simulink model "TTR_mdl"  (Simulink 8.1)
settings: Solver=ode3  StartTime=0.0  StopTime=100  FixedStep=Ts  MaxStep=Ts  RelTol=1e-3
InitFcn:
  | TTR_mdl_Initialization;
model workspace: external: MAT-File C:\Users\Kostas\Documents\GitHub\robust_mpc\Verified_Examples\TTR\TTR_mdl_workspace.mat (data not in the file)
values from neighbouring files (symbols this model uses):
  Damping = [damping_phi; damping_theta; damping_psi; damping_x; damping_y; damping_z]    [TTR_Initialization.m]    (also in TTR_mdl_Dynamics.m = block.DialogPrm(3).Data; TTR_mdl_Initialization.m = cell2struct( num2cell(Damping_arr), {'phi','theta','psi','x'; TTR_mdl_workspace.mat = )
  Drag = block.DialogPrm(4).Data    [TTR_mdl_Dynamics.m]    (also in TTR_mdl_Initialization.m = cell2struct( num2cell(Drag_arr), {'a','b'}, 1 ); TTR_mdl_workspace.mat = )
  F_0 = block.DialogPrm(5).Data    [TTR_mdl_Dynamics.m]    (also in TTR_mdl_Initialization.m = solve('d_RL_x*(FL_0+FR_0)=d_T_x*FT_0','FR_0+FL_0+FT_0=m_B*g'; TTR_mdl_workspace.mat = )
  g = 9.81    [TTR_Initialization.m]    (also in TTR_mdl_Dynamics.m = TTR_mdl_Properties.g; TTR_mdl_Initialization.m)
  LQR_phi = [92.7047477254 36.0877897074 4.11128151093 0.0597844255793]    [TTR_mdl_workspace.mat]
  m_B = 2.350    (= 2.35)    [TTR_Initialization.m]    (also in TTR_mdl_Dynamics.m = TTR_mdl_Properties.m_B; TTR_mdl_Initialization.m)
  PolyGT_U2A = [0.002181661564993 0.0]    [TTR_Initialization.m]    (also in TTR_mdl_Initialization.m; TTR_mdl_workspace.mat = [0.00218166156499 0])
  PolyRL_U2R = (PolyR_U2R + PolyL_U2R)/2    [TTR_mdl_Initialization.m]    (also in TTR_mdl_workspace.mat = [7.59051955434 1446.30527598])
  PolyT_U2R = 1.0e+03*[0.007882307894585   1.022799157396815]    [TTR_Initialization.m]    (also in TTR_mdl_Initialization.m; TTR_mdl_workspace.mat = [7.88230789458 1022.7991574])
  Rotor_Properties = cell2struct( num2cell(Rotor_Properties_arr), {'C_T_RL_trim','C_T_RL_prop','C_T_T_trim','C_T_T_prop'}, 1 )    [TTR_mdl_Initialization.m]    (also in TTR_mdl_workspace.mat = )
  tf_RL0_ss = idss(tf_RL0_p,'SSParameterization','Canonical')    [TTR_mdl_Initialization.m]
  tf_RL_ss = idss(tf_RL_p,'SSParameterization','Canonical')    [TTR_mdl_Initialization.m]
  tf_S_den = tf_S.den{1}    [TTR_mdl_Initialization.m]    (also in TTR_mdl_workspace.mat = [1 30])
  tf_S_num = tf_S.num{1}    [TTR_mdl_Initialization.m]    (also in TTR_mdl_workspace.mat = [0 30])
  tf_T0_ss = idss(tf_T0_p,'SSParameterization','Canonical')    [TTR_mdl_Initialization.m]
  tf_T_ss = idss(tf_T_p,'SSParameterization','Canonical')    [TTR_mdl_Initialization.m]
  Ts_slow = 0.250    (= 0.25)    [TTR_Initialization.m]    (also in TTR_mdl_Initialization.m = TTR_RobustMPC.Xdir.Ts; TTR_mdl_workspace.mat = 0.2)
  TTR_mdl_Properties = block.DialogPrm(1).Data    [TTR_mdl_Dynamics.m]    (also in TTR_mdl_Initialization.m = cell2struct( num2cell(TTR_mdl_Properties_arr), {'m_B','g','I; TTR_mdl_workspace.mat = )
  TTR_mdl_Properties_arr = [ m_B; g; Ixx; Iyy; Izz; Ixy; Ixz; Iyz; d_RL_x; d_T_x; d_RL_y; d_T_y; d_RL_z; d_T_z; h_RL; h_T; rho; w_chord; w_span; w_ac_x; w_ac_y ]    [TTR_mdl_Initialization.m]    (also in TTR_mdl_workspace.mat = [2.35 9.81 0.057748141 0.025379458 0.074710979 0 0 0 0.05461)
  TTR_RobustMPC =     [RobustMPC_TTRctrls.mat]    (also in RobustMPC_TTRctrls_INFnorm.mat)
  Wing_Properties = block.DialogPrm(2).Data    [TTR_mdl_Dynamics.m]    (also in TTR_mdl_Initialization.m = struct(                  'a_vect' , a_vect ,                ; TTR_mdl_workspace.mat = )
libraries: simulink_extras x5, Robust_MPC_Library x3
settings Model: Creator=babis  LastModifiedBy=Kostas
settings SolverCC: AutoInsertRateTranBlk=on  InsertRTBMode=Always
settings DataIOCC: SaveOutput=off  SaveState=on
settings OptimizationCC: InlineParams=on  InlineInvariantSignals=on  StateBitsets=on  DataBitsets=on  UseTempVars=on  ZeroExternalMemoryAtStartup=off  ZeroInternalMemoryAtStartup=off  NoFixptDivByZeroProtection=on  OptimizeModelRefInitCode=on  LifeSpan=1
settings DebuggingCC: AlgebraicLoopMsg=none  SolverPrmCheckMsg=none  UnconnectedInputMsg=none  UnconnectedOutputMsg=none  UnconnectedLineMsg=none
settings HardwareCC: ProdIntDivRoundTo=Floor  ProdEndianess=LittleEndian  ProdHWDeviceType=Generic->Custom
settings SFSimCC: SimUserIncludeDirs=/home/atum/workspace/Matlab/src  SimBuildMode=sf_nonincremental_build
settings RTWCC: SystemTargetFile=ert.tlc  TLCOptions=-p0  GenCodeOnly=on  TemplateMakefile=ert_default_tmf  Description=Real-Time Workshop Embedded Coder  GenerateReport=on  RTWVerbose=off  ProcessScript=ert_make_rtw_hook  RTWUseSimCustomCode=on  CustomInclude=/home/atum/workspace/Matlab/src  IncludeHyperlinkInReport=on  LaunchReport=on
settings CodeAppCC: ForceParamTrailComments=on  IgnoreCustomStorageClasses=off  SimulinkDataObjDesc=on  CustomSymbolStrGlobalVar=rt$N$M  CustomSymbolStrType=$N$M  CustomSymbolStrFcn=$N$M$F  CustomSymbolStrMacro=$N$M  InsertBlockDesc=on  InternalIdentifier=Classic
settings ERTTargetCC: CodeReplacementLibrary=ISO_C  MultiwordLength=2048  GenerateSampleERTMain=on  IncludeMdlTerminateFcn=off  SuppressErrorStatus=on  SupportAbsoluteTime=off  SupportNonFinite=off  SupportComplex=off  InlinedParameterPlacement=NonHierarchical  RootIOFormat=Structure reference  ERTCustomFileTemplate=example_file_process.tlc  ConvertIfToSwitch=off  SuppressUnreachableDefaultCases=off

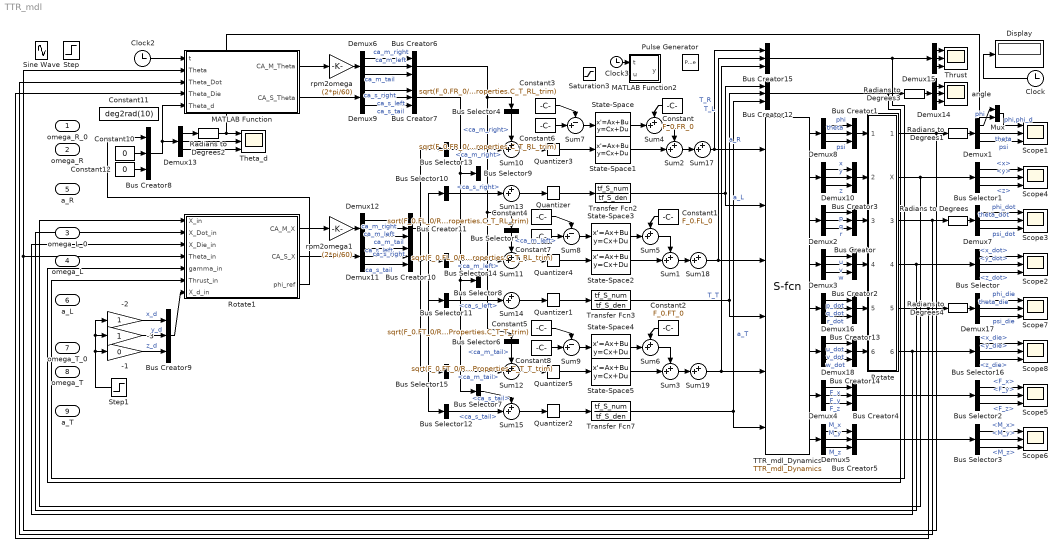
== system TTR_mdl ==
  omega_R_0 : Inport
  omega_R : Inport  Port=2
  omega_L_0 : Inport  Port=3
  omega_L : Inport  Port=4
  a_R : Inport  Port=5
  a_L : Inport  Port=6
  omega_T_0 : Inport  Port=7
  omega_T : Inport  Port=8
  a_T : Inport  Port=9
  -1 : Gain  Gain=0
  -2 : Gain
  -3 : Gain
  Bus Creator{,1..15} (16 alike) : BusCreator  Inputs=3
  Bus Selector : BusSelector  OutputSignals=x_dot,y_dot,z_dot
  Bus Selector1 : BusSelector  OutputSignals=x,y,z
  Bus Selector10 : BusSelector  OutputSignals=ca_s_right
  Bus Selector11 : BusSelector  OutputSignals=ca_s_left
  Bus Selector12 : BusSelector  OutputSignals=ca_s_tail
  Bus Selector13 : BusSelector  OutputSignals=ca_m_right
  Bus Selector14 : BusSelector  OutputSignals=ca_m_left
  Bus Selector15 : BusSelector  OutputSignals=ca_m_tail
  Bus Selector16 : BusSelector  OutputSignals=x_die,y_die,z_die
  Bus Selector2 : BusSelector  OutputSignals=F_x,F_y,F_z
  Bus Selector3 : BusSelector  OutputSignals=M_x,M_y,M_z
  Bus Selector4 : BusSelector  OutputSignals=ca_m_right
  Bus Selector5 : BusSelector  OutputSignals=ca_m_left
  Bus Selector6 : BusSelector  OutputSignals=ca_m_tail
  Bus Selector7 : BusSelector  OutputSignals=ca_s_tail
  Bus Selector8 : BusSelector  OutputSignals=ca_s_left
  Bus Selector9 : BusSelector  OutputSignals=ca_s_right
  Clock : Clock
  Clock2 : Clock
  Clock3 : Clock
  Constant : Constant  Value=F_0.FR_0
  Constant1 : Constant  Value=F_0.FL_0
  Constant10 : Constant  Value=0
  Constant11 : Constant  Value=deg2rad(10)
  Constant12 : Constant  Value=0
  Constant2 : Constant  Value=F_0.FT_0
  Constant3 : Constant  Value=sqrt(F_0.FR_0/Rotor_Properties.C_T_RL_trim)
  Constant4 : Constant  Value=sqrt(F_0.FL_0/Rotor_Properties.C_T_RL_trim)
  Constant5 : Constant  Value=sqrt(F_0.FT_0/Rotor_Properties.C_T_T_trim)
  Constant6 : Constant  Value=sqrt(F_0.FR_0/Rotor_Properties.C_T_RL_trim)
  Constant7 : Constant  Value=sqrt(F_0.FL_0/Rotor_Properties.C_T_RL_trim)
  Constant8 : Constant  Value=sqrt(F_0.FT_0/Rotor_Properties.C_T_T_trim)
  Demux{1..18} (18 alike) : Demux  Outputs=3
  Display : Display
  MATLAB Function : MATLAB Function  TreatAsAtomicUnit=on
  MATLAB Function2 : MATLAB Function  TreatAsAtomicUnit=on
  Mux : Mux  Inputs=2
  Pulse Generator : DiscretePulseGenerator  PulseType=Time based  Amplitude=0.1  Period=10  PulseWidth=50
  Quantizer : Quantizer  QuantizationInterval=deg2rad(0.5)
  Quantizer1 : Quantizer  QuantizationInterval=deg2rad(0.5)
  Quantizer2 : Quantizer  QuantizationInterval=deg2rad(0.5)
  Quantizer3 : Quantizer  QuantizationInterval=(1/(2*pi/60))*(1/PolyRL_U2R(1))
  Quantizer4 : Quantizer  QuantizationInterval=(1/(2*pi/60))*(1/PolyRL_U2R(1))
  Quantizer5 : Quantizer  QuantizationInterval=(1/(2*pi/60))*(1/PolyT_U2R(1))
  Radians to Degrees{,1..4} (5 alike) : simulink_extras/Transformations/Radians to Degrees
  Rotate : Subsystem
  Rotate1 : Subsystem
  Saturation3 : Saturate  UpperLimit=deg2rad(15)  LowerLimit=-deg2rad(15)
  Scope{1..8} (8 alike) : Scope  NumInputPorts=3
      Scope1 settings: TimeRange=100  YMin=-3.5~-0.225~-0.05  YMax=3.5~0.35~0.225  SaveName=Theta
      Scope2 settings: TimeRange=100  YMin=-0.004~0.005~0.0255  YMax=0.003~0.025~0.0285  SaveName=X_Dot
      Scope3 settings: TimeRange=100  YMin=-45~-0.25~-0.06  YMax=-30~0.25~0.02  SaveName=Theta_Dot
      Scope4 settings: TimeRange=100  YMin=5.55112e-17~0.1~-0.0225  YMax=1.5~2~0.015  SaveName=X
      Scope5 settings: TimeRange=100  YMin=-1~-2~-0.8  YMax=2.5~3~0.6000000000000001  SaveName=F
      Scope6 settings: TimeRange=100  YMin=-0.1~-0.01~-0.015  YMax=0.1~0.015~0.01  SaveName=M
      Scope7 settings: TimeRange=100  YMin=-100~-30~-10  YMax=100~30~10  SaveName=Theta_Die
      Scope8 settings: TimeRange=100  YMin=0~0~-5  YMax=100~800~5  SaveName=X_Die
  Sine Wave : Sin  Amplitude=deg2rad(10)  Frequency=0.1*(60/(2*pi))  SampleTime=0
  State-Space : StateSpace  A=tf_RL0_ss.A  B=tf_RL0_ss.B  C=tf_RL0_ss.C  D=tf_RL0_ss.D  X0=[0;0]
  State-Space1 : StateSpace  A=tf_RL_ss.A  B=tf_RL_ss.B  C=tf_RL_ss.C  D=tf_RL_ss.D  X0=[0;0]
  State-Space2 : StateSpace  A=tf_RL_ss.A  B=tf_RL_ss.B  C=tf_RL_ss.C  D=tf_RL_ss.D  X0=[0;0]
  State-Space3 : StateSpace  A=tf_RL0_ss.A  B=tf_RL0_ss.B  C=tf_RL0_ss.C  D=tf_RL0_ss.D  X0=[0;0]
  State-Space4 : StateSpace  A=tf_T0_ss.A  B=tf_T0_ss.B  C=tf_T0_ss.C  D=tf_T0_ss.D  X0=[0;0]
  State-Space5 : StateSpace  A=tf_T_ss.A  B=tf_T_ss.B  C=tf_T_ss.C  D=tf_T_ss.D  X0=[0;0]
  Step : Step  Time=50  After=[-1;-1;1]  SampleTime=0
  Step1 : Step  SampleTime=0
  Sum{1..6,10..15,17..19} (15 alike) : Sum  Inputs=++|
  Sum7 : Sum  Inputs=-+|
  Sum8 : Sum  Inputs=-+|
  Sum9 : Sum  Inputs=-+|
  TTR_mdl_Dynamics : M-S-Function  FunctionName=TTR_mdl_Dynamics  Parameters=TTR_mdl_Properties,Wing_Properties,Damping,Drag,F_0  mask{TTR_mdl_Properties=TTR_mdl_Properties, Wing_Properties=Wing_Properties, Damping=Damping, Drag=Drag, F_0=F_0}
      mask Display:
      | port_label('input',1,'T_R')
      | port_label('input',2,'a_R')
      | port_label('input',3,'T_L')
      | port_label('input',4,'a_L')
      | port_label('input',5,'T_T')
      | port_label('input',6,'a_T')
      | 
      | port_label('output',1,'Theta')
      | port_label('output',2,'X')
      | port_label('output',3,'Omega')
      | port_label('output',4,'U')
      | 
      | port_label('output',5,'Omega_Dot')
      | port_label('output',6,'U_Dot')
      | 
      | port_label('output',7,'F_tot')
      | port_label('output',8,'M_tot')
  Theta_d : Scope  NumInputPorts=3
      settings: TimeRange=100  YMin=0.248709~-9525~-5  YMax=0.274889~-9300~5  SaveName=Theta_d
  Thrust : Scope  NumInputPorts=3
      settings: TimeRange=16  YMin=10.2759~10.2759~1.516  YMax=11.3575~11.3575~1.529  SaveName=F_A
  Transfer Fcn2 : TransferFcn  Numerator=tf_S_num  Denominator=tf_S_den
  Transfer Fcn3 : TransferFcn  Numerator=tf_S_num  Denominator=tf_S_den
  Transfer Fcn7 : TransferFcn  Numerator=tf_S_num  Denominator=tf_S_den
  angle : Scope  NumInputPorts=3
      settings: TimeRange=100  YMin=14.25~14.25~-1  YMax=15.75~15.75~1  SaveName=Gamma
  rpm2omega : Gain  Gain=(2*pi/60)
  rpm2omega1 : Gain  Gain=(2*pi/60)
  wires:
  Transfer Fcn2/1 -> TTR_mdl_Dynamics/2, Bus Creator12/1  "a_R"
  Transfer Fcn3/1 -> TTR_mdl_Dynamics/4, Bus Creator12/2  "a_L"
  Radians to Degrees/1 -> Demux7/1
  Clock/1 -> Display/1
  Demux7/1 -> Scope3/1  "phi_dot"
  Demux7/2 -> Scope3/2  "theta_dot"
  Demux7/3 -> Scope3/3  "psi_dot"
  Radians to Degrees1/1 -> Demux1/1
  Demux1/2 -> Scope1/2  "theta"
  Demux1/3 -> Scope1/3  "psi"
  Bus Selector1/1 -> Scope4/1  "<x>"
  Bus Selector1/2 -> Scope4/2  "<y>"
  Bus Selector1/3 -> Scope4/3  "<z>"
  Bus Selector3/1 -> Scope6/1  "<M_x>"
  Bus Selector3/2 -> Scope6/2  "<M_y>"
  Bus Selector3/3 -> Scope6/3  "<M_z>"
  Transfer Fcn7/1 -> TTR_mdl_Dynamics/6, Bus Creator12/3  "a_T"
  State-Space1/1 -> Sum2/2
  State-Space2/1 -> Sum1/2
  State-Space5/1 -> Sum3/2
  State-Space/1 -> Sum4/2
  Sum4/1 -> Sum2/1
  Constant/1 -> Sum4/1
  Constant1/1 -> Sum5/1
  State-Space3/1 -> Sum5/2
  Sum5/1 -> Sum1/1
  Constant2/1 -> Sum6/1
  State-Space4/1 -> Sum6/2
  Sum6/1 -> Sum3/1
  Sum7/1 -> State-Space/1
  Constant3/1 -> Sum7/1
  Constant4/1 -> Sum8/1
  Sum8/1 -> State-Space3/1
  Constant5/1 -> Sum9/1
  Sum9/1 -> State-Space4/1
  Constant6/1 -> Sum7/2
  Constant7/1 -> Sum8/2
  Constant8/1 -> Sum9/2
  Demux2/1 -> Bus Creator/1  "p"
  Demux2/2 -> Bus Creator/2  "q"
  Demux2/3 -> Bus Creator/3  "r"
  Demux8/1 -> Bus Creator1/1  "phi"
  Demux8/2 -> Bus Creator1/2  "theta"
  Demux8/3 -> Bus Creator1/3  "psi"
  Demux3/1 -> Bus Creator2/1  "u"
  Demux3/2 -> Bus Creator2/2  "v"
  Demux3/3 -> Bus Creator2/3  "w"
  Demux10/1 -> Bus Creator3/1  "x"
  Demux10/2 -> Bus Creator3/2  "y"
  Bus Selector/1 -> Scope2/1  "<x_dot>"
  Bus Selector/2 -> Scope2/2  "<y_dot>"
  Bus Selector/3 -> Scope2/3  "<z_dot>"
  Demux4/1 -> Bus Creator4/1  "F_x"
  Demux4/2 -> Bus Creator4/2  "F_y"
  Demux4/3 -> Bus Creator4/3  "F_z"
  Bus Creator4/1 -> Bus Selector2/1
  Bus Selector2/1 -> Scope5/1  "<F_x>"
  Bus Selector2/2 -> Scope5/2  "<F_y>"
  Bus Selector2/3 -> Scope5/3  "<F_z>"
  Demux5/1 -> Bus Creator5/1  "M_x"
  Demux5/2 -> Bus Creator5/2  "M_y"
  Demux5/3 -> Bus Creator5/3  "M_z"
  Bus Creator5/1 -> Bus Selector3/1
  Demux6/1 -> Bus Creator6/1  "ca_m_right"
  Demux6/2 -> Bus Creator6/2  "ca_m_left"
  Demux6/3 -> Bus Creator6/3  "ca_m_tail"
  Sum10/1 -> Quantizer3/1
  Sum11/1 -> Quantizer4/1
  Sum12/1 -> Quantizer5/1
  MATLAB Function/1(CA_M_Theta) -> rpm2omega/1
  rpm2omega/1 -> Demux6/1
  Demux9/1 -> Bus Creator7/1  "ca_s_right"
  Demux9/2 -> Bus Creator7/2  "ca_s_left"
  Demux9/3 -> Bus Creator7/3  "ca_s_tail"
  MATLAB Function/2(CA_S_Theta) -> Demux9/1
  Bus Creator6/1 -> Bus Selector5/1, Bus Selector6/1, Bus Selector4/1
  Bus Selector4/1 -> Sum10/1  "<ca_m_right>"
  Bus Selector5/1 -> Sum11/1  "<ca_m_left>"
  Bus Selector6/1 -> Sum12/1  "<ca_m_tail>"
  Sum14/1 -> Quantizer1/1
  Sum15/1 -> Quantizer2/1
  Bus Selector7/1 -> Sum15/1  "<ca_s_tail>"
  Bus Creator7/1 -> Bus Selector7/1, Bus Selector8/1, Bus Selector9/1
  Constant12/1 -> Bus Creator8/3
  Demux11/2 -> Bus Creator10/2  "ca_s_left"
  Demux11/3 -> Bus Creator10/3  "ca_s_tail"
  Demux12/1 -> Bus Creator11/1  "ca_m_right"
  Demux12/2 -> Bus Creator11/2  "ca_m_left"
  Demux12/3 -> Bus Creator11/3  "ca_m_tail"
  Demux11/1 -> Bus Creator10/1  "ca_s_right"
  Bus Creator10/1 -> Bus Selector10/1, Bus Selector11/1, Bus Selector12/1
  Clock2/1 -> MATLAB Function/1(t)
  Bus Creator11/1 -> Bus Selector13/1, Bus Selector14/1, Bus Selector15/1
  Sum13/1 -> Quantizer/1
  Clock3/1 -> MATLAB Function2/1(t)
  Bus Creator8/1 -> MATLAB Function/5(Theta_d), Demux13/1
  Constant10/1 -> Bus Creator8/2
  Demux13/1 -> Radians to Degrees2/1
  Demux13/2 -> Theta_d/2
  Demux13/3 -> Theta_d/3
  Demux14/1 -> angle/1
  Demux14/2 -> angle/2
  Demux14/3 -> angle/3
  Bus Creator12/1 -> Radians to Degrees3/1, Rotate1/5(gamma_in)
  Radians to Degrees3/1 -> Demux14/1
  TTR_mdl_Dynamics/8 -> Demux5/1
  TTR_mdl_Dynamics/7 -> Demux4/1
  TTR_mdl_Dynamics/1 -> Demux8/1
  TTR_mdl_Dynamics/2 -> Demux10/1
  TTR_mdl_Dynamics/4 -> Demux3/1
  TTR_mdl_Dynamics/3 -> Demux2/1
  Radians to Degrees4/1 -> Demux17/1
  Demux17/1 -> Scope7/1  "phi_die"
  Demux17/2 -> Scope7/2  "theta_die"
  Demux17/3 -> Scope7/3  "psi_die"
  Demux16/1 -> Bus Creator13/1  "p_dot"
  Demux16/2 -> Bus Creator13/2  "q_dot"
  Demux16/3 -> Bus Creator13/3  "r_dot"
  TTR_mdl_Dynamics/5 -> Demux16/1
  Bus Selector16/1 -> Scope8/1  "<x_die>"
  Bus Selector16/2 -> Scope8/2  "<y_die>"
  Bus Selector16/3 -> Scope8/3  "<z_die>"
  TTR_mdl_Dynamics/6 -> Demux18/1
  Demux18/1 -> Bus Creator14/1  "u_dot"
  Demux18/2 -> Bus Creator14/2  "v_dot"
  Demux18/3 -> Bus Creator14/3  "w_dot"
  Bus Selector13/1 -> Sum10/2  "<ca_m_right>"
  Bus Selector10/1 -> Sum13/2  "<ca_s_right>"
  Bus Selector14/1 -> Sum11/2  "<ca_m_left>"
  Bus Selector11/1 -> Sum14/2  "<ca_s_left>"
  Bus Selector15/1 -> Sum12/2  "<ca_m_tail>"
  Bus Selector12/1 -> Sum15/2  "<ca_s_tail>"
  Step1/1 -> -2/1, -3/1, -1/1
  rpm2omega1/1 -> Demux12/1
  -1/1 -> Bus Creator9/3  "z_d"
  Sum2/1 -> Sum17/2
  Sum17/1 -> TTR_mdl_Dynamics/1, Bus Creator15/1  "T_R"
  Sum1/1 -> Sum18/2
  Sum18/1 -> TTR_mdl_Dynamics/3, Bus Creator15/2  "T_L"
  Sum3/1 -> Sum19/2
  Sum19/1 -> TTR_mdl_Dynamics/5, Bus Creator15/3  "T_T"
  Demux1/1 -> Mux/1  "phi"
  Mux/1 -> Scope1/1  "phi,phi_d"
  Bus Creator1/1 -> Rotate/1(Theta_in)
  Bus Creator3/1 -> Rotate/2(X_in)
  Bus Creator/1 -> Rotate/3(Omega_in)
  Bus Creator2/1 -> Rotate/4(U_in)
  Bus Creator13/1 -> Rotate/5(Omega_Dot_in)
  Bus Creator14/1 -> Rotate/6(U_Dot_in)
  Rotate/1(Theta) -> Radians to Degrees1/1, MATLAB Function/2(Theta), Rotate1/4(Theta_in)
  Rotate/2(X) -> Bus Selector1/1, Rotate1/1(X_in)
  Rotate/3(Theta_Dot) -> Radians to Degrees/1, MATLAB Function/3(Theta_Dot)
  Rotate/4(X_Dot) -> Bus Selector/1, Rotate1/2(X_Dot_in)
  Rotate/5(Theta_Die) -> Radians to Degrees4/1, MATLAB Function/4(Theta_Die)
  Rotate/6(X_Die) -> Bus Selector16/1, Rotate1/3(X_Die_in)
  Quantizer1/1 -> Transfer Fcn3/1
  Quantizer2/1 -> Transfer Fcn7/1
  Quantizer/1 -> Transfer Fcn2/1
  Quantizer3/1 -> State-Space1/1
  Quantizer4/1 -> State-Space2/1
  Quantizer5/1 -> State-Space5/1
  -2/1 -> Bus Creator9/1  "x_d"
  -3/1 -> Bus Creator9/2  "y_d"
  Demux10/3 -> Bus Creator3/3  "z"
  Radians to Degrees2/1 -> Theta_d/1, Mux/2
  Bus Creator9/1 -> Rotate1/7(X_d_in)
  Rotate1/1(CA_M_X) -> rpm2omega1/1
  Rotate1/2(CA_S_X) -> Demux11/1
  Rotate1/3(phi_ref) -> Bus Creator8/1
  Demux15/1 -> Thrust/1
  Demux15/2 -> Thrust/2
  Demux15/3 -> Thrust/3
  Bus Creator15/1 -> Demux15/1, Rotate1/6(Thrust_in)

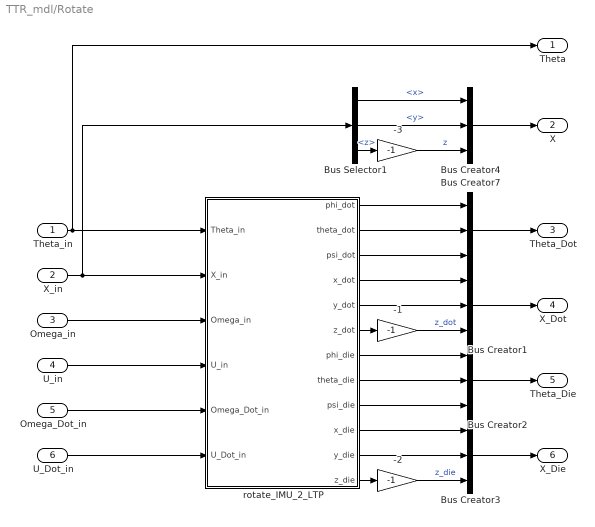
== system TTR_mdl/Rotate ==
  Theta_in : Inport
  X_in : Inport  Port=2
  Omega_in : Inport  Port=3
  U_in : Inport  Port=4
  Omega_Dot_in : Inport  Port=5
  U_Dot_in : Inport  Port=6
  -1 : Gain  Gain=-1
  -2 : Gain  Gain=-1
  -3 : Gain  Gain=-1
  Bus Creator{1..4,7} (5 alike) : BusCreator  Inputs=3
  Bus Selector1 : BusSelector  OutputSignals=x,y,z
  rotate_IMU_2_LTP : MATLAB Function  TreatAsAtomicUnit=on
  Theta : Outport
  X : Outport  Port=2
  Theta_Dot : Outport  Port=3
  X_Dot : Outport  Port=4
  Theta_Die : Outport  Port=5
  X_Die : Outport  Port=6
  wires:
  Theta_in/1 -> Theta/1, rotate_IMU_2_LTP/1(Theta_in)
  X_in/1 -> rotate_IMU_2_LTP/2(X_in), Bus Selector1/1
  Omega_in/1 -> rotate_IMU_2_LTP/3(Omega_in)
  U_in/1 -> rotate_IMU_2_LTP/4(U_in)
  Omega_Dot_in/1 -> rotate_IMU_2_LTP/5(Omega_Dot_in)
  U_Dot_in/1 -> rotate_IMU_2_LTP/6(U_Dot_in)
  rotate_IMU_2_LTP/1(phi_dot) -> Bus Creator7/1
  rotate_IMU_2_LTP/2(theta_dot) -> Bus Creator7/2
  rotate_IMU_2_LTP/3(psi_dot) -> Bus Creator7/3
  rotate_IMU_2_LTP/4(x_dot) -> Bus Creator1/1
  rotate_IMU_2_LTP/5(y_dot) -> Bus Creator1/2
  rotate_IMU_2_LTP/6(z_dot) -> -1/1
  rotate_IMU_2_LTP/7(phi_die) -> Bus Creator2/1
  rotate_IMU_2_LTP/8(theta_die) -> Bus Creator2/2
  rotate_IMU_2_LTP/9(psi_die) -> Bus Creator2/3
  rotate_IMU_2_LTP/10(x_die) -> Bus Creator3/1
  rotate_IMU_2_LTP/11(y_die) -> Bus Creator3/2
  rotate_IMU_2_LTP/12(z_die) -> -2/1
  Bus Creator7/1 -> Theta_Dot/1
  Bus Creator1/1 -> X_Dot/1
  Bus Creator2/1 -> Theta_Die/1
  Bus Creator3/1 -> X_Die/1
  -1/1 -> Bus Creator1/3  "z_dot"
  -2/1 -> Bus Creator3/3  "z_die"
  Bus Creator4/1 -> X/1
  Bus Selector1/1 -> Bus Creator4/1  "<x>"
  Bus Selector1/2 -> Bus Creator4/2  "<y>"
  Bus Selector1/3 -> -3/1  "<z>"
  -3/1 -> Bus Creator4/3  "z"

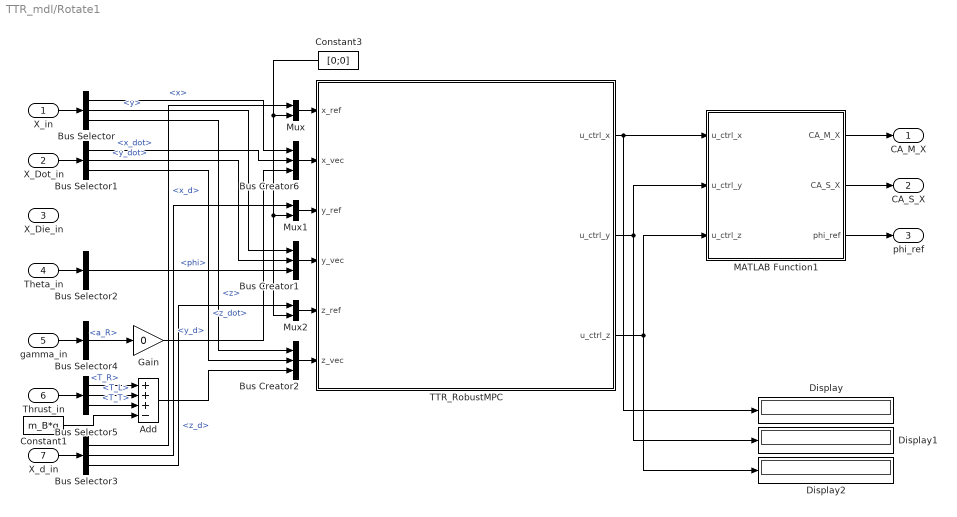
== system TTR_mdl/Rotate1 ==
  X_in : Inport
  X_Dot_in : Inport  Port=2
  X_Die_in : Inport  Port=3
  Theta_in : Inport  Port=4
  gamma_in : Inport  Port=5
  Thrust_in : Inport  Port=6
  X_d_in : Inport  Port=7
  Add : Sum  Inputs=+++-
  Bus Creator1 : BusCreator  Inputs=3
  Bus Creator2 : BusCreator  Inputs=3
  Bus Creator6 : BusCreator  Inputs=3
  Bus Selector : BusSelector  OutputSignals=x,y,z
  Bus Selector1 : BusSelector  OutputSignals=x_dot,y_dot,z_dot
  Bus Selector2 : BusSelector  OutputSignals=phi
  Bus Selector3 : BusSelector  OutputSignals=x_d,y_d,z_d
  Bus Selector4 : BusSelector  OutputSignals=a_R
  Bus Selector5 : BusSelector  OutputSignals=T_R,T_L,T_T
  Constant1 : Constant  Value=m_B*g
  Constant3 : Constant  Value=[0;0]
  Display : Display
  Display1 : Display
  Display2 : Display
  Gain : Gain  Gain=0
  MATLAB Function1 : MATLAB Function  TreatAsAtomicUnit=on
  Mux : Mux  Inputs=2
  Mux1 : Mux  Inputs=2
  Mux2 : Mux  Inputs=2
  TTR_RobustMPC : Subsystem
  CA_M_X : Outport
  CA_S_X : Outport  Port=2
  phi_ref : Outport  Port=3
  wires:
  TTR_RobustMPC/2(u_ctrl_y) -> Display1/1, MATLAB Function1/2(u_ctrl_y)
  TTR_RobustMPC/3(u_ctrl_z) -> Display2/1, MATLAB Function1/3(u_ctrl_z)
  X_in/1 -> Bus Selector/1
  X_Dot_in/1 -> Bus Selector1/1
  Theta_in/1 -> Bus Selector2/1
  Bus Creator6/1 -> TTR_RobustMPC/2(x_vec)
  Bus Selector/1 -> Bus Creator6/1  "<x>"
  Bus Selector1/1 -> Bus Creator6/2  "<x_dot>"
  gamma_in/1 -> Bus Selector4/1
  Bus Creator1/1 -> TTR_RobustMPC/4(y_vec)
  Bus Selector/2 -> Bus Creator1/1  "<y>"
  Bus Selector1/2 -> Bus Creator1/2  "<y_dot>"
  Bus Selector2/1 -> Bus Creator1/3  "<phi>"
  Bus Creator2/1 -> TTR_RobustMPC/6(z_vec)
  Bus Selector/3 -> Bus Creator2/1  "<z>"
  Bus Selector1/3 -> Bus Creator2/2  "<z_dot>"
  TTR_RobustMPC/1(u_ctrl_x) -> MATLAB Function1/1(u_ctrl_x), Display/1
  MATLAB Function1/1(CA_M_X) -> CA_M_X/1
  MATLAB Function1/2(CA_S_X) -> CA_S_X/1
  MATLAB Function1/3(phi_ref) -> phi_ref/1
  Mux/1 -> TTR_RobustMPC/1(x_ref)
  Mux1/1 -> TTR_RobustMPC/3(y_ref)
  Mux2/1 -> TTR_RobustMPC/5(z_ref)
  Constant3/1 -> Mux/2, Mux1/2, Mux2/2
  X_d_in/1 -> Bus Selector3/1
  Bus Selector3/1 -> Mux/1  "<x_d>"
  Bus Selector3/2 -> Mux1/1  "<y_d>"
  Bus Selector3/3 -> Mux2/1  "<z_d>"
  Bus Selector4/1 -> Gain/1  "<a_R>"
  Thrust_in/1 -> Bus Selector5/1
  Bus Selector5/1 -> Add/1  "<T_R>"
  Bus Selector5/2 -> Add/2  "<T_L>"
  Bus Selector5/3 -> Add/3  "<T_T>"
  Add/1 -> Bus Creator2/3
  Constant1/1 -> Add/4
  Gain/1 -> Bus Creator6/3

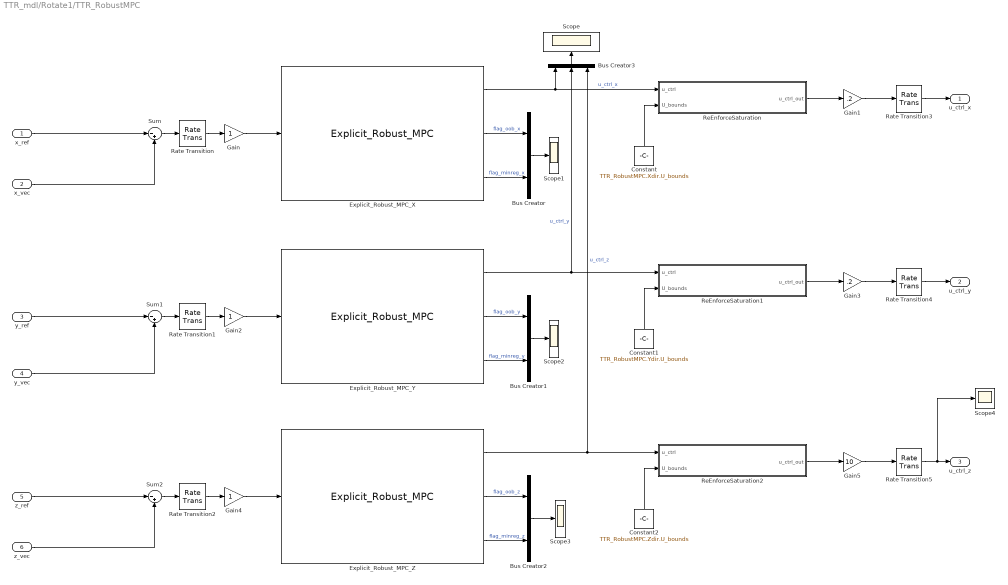
== system TTR_mdl/Rotate1/TTR_RobustMPC ==
  x_ref : Inport
  x_vec : Inport  Port=2
  y_ref : Inport  Port=3
  y_vec : Inport  Port=4
  z_ref : Inport  Port=5
  z_vec : Inport  Port=6
  Bus Creator : BusCreator  Inputs=2
  Bus Creator1 : BusCreator  Inputs=2
  Bus Creator2 : BusCreator  Inputs=2
  Bus Creator3 : BusCreator  Inputs=3
  Constant : Constant  Value=TTR_RobustMPC.Xdir.U_bounds
  Constant1 : Constant  Value=TTR_RobustMPC.Ydir.U_bounds
  Constant2 : Constant  Value=TTR_RobustMPC.Zdir.U_bounds
  Explicit_Robust_MPC_X : Robust_MPC_Library/Explicit_Robust_MPC  H=TTR_RobustMPC.Xdir.H  K=TTR_RobustMPC.Xdir.K  F=TTR_RobustMPC.Xdir.F  G=TTR_RobustMPC.Xdir.G  Nc=TTR_RobustMPC.Xdir.Nc  Nx=TTR_RobustMPC.Xdir.Nx  Hi_init=zeros(100,TTR_RobustMPC.Xdir.Nx)  Ki_init=zeros(100,TTR_RobustMPC.Xdir.Nu)
  Explicit_Robust_MPC_Y : Robust_MPC_Library/Explicit_Robust_MPC  H=TTR_RobustMPC.Ydir.H  K=TTR_RobustMPC.Ydir.K  F=TTR_RobustMPC.Ydir.F  G=TTR_RobustMPC.Ydir.G  Nc=TTR_RobustMPC.Ydir.Nc  Nx=TTR_RobustMPC.Ydir.Nx  Hi_init=zeros(100,TTR_RobustMPC.Ydir.Nx)  Ki_init=zeros(100,TTR_RobustMPC.Ydir.Nu)
  Explicit_Robust_MPC_Z : Robust_MPC_Library/Explicit_Robust_MPC  H=TTR_RobustMPC.Zdir.H  K=TTR_RobustMPC.Zdir.K  F=TTR_RobustMPC.Zdir.F  G=TTR_RobustMPC.Zdir.G  Nc=TTR_RobustMPC.Zdir.Nc  Nx=TTR_RobustMPC.Zdir.Nx  Hi_init=zeros(100,TTR_RobustMPC.Zdir.Nx)  Ki_init=zeros(100,TTR_RobustMPC.Zdir.Nu)
  Gain : Gain  SampleTime=TTR_RobustMPC.Xdir.Ts
  Gain1 : Gain  Gain=.2  SampleTime=TTR_RobustMPC.Xdir.Ts
  Gain2 : Gain  SampleTime=TTR_RobustMPC.Ydir.Ts
  Gain3 : Gain  Gain=.2  SampleTime=TTR_RobustMPC.Ydir.Ts
  Gain4 : Gain  SampleTime=TTR_RobustMPC.Zdir.Ts
  Gain5 : Gain  Gain=10  SampleTime=TTR_RobustMPC.Zdir.Ts
  Rate Transition{,1..5} (6 alike) : RateTransition
  ReEnforceSaturation : MATLAB Function  TreatAsAtomicUnit=on
  ReEnforceSaturation1 : MATLAB Function  TreatAsAtomicUnit=on
  ReEnforceSaturation2 : MATLAB Function  TreatAsAtomicUnit=on
  Scope{,1..4} (5 alike) : Scope
      Scope settings: SaveName=RobustMPC_uctrl_xyz
      Scope3 settings: SaveName=ScopeData2
      Scope4 settings: YMin=-0.1  YMax=1.2  SaveName=ScopeData3
  Sum : Sum  Inputs=|-+
  Sum1 : Sum  Inputs=|-+
  Sum2 : Sum  Inputs=|-+
  u_ctrl_x : Outport
  u_ctrl_y : Outport  Port=2
  u_ctrl_z : Outport  Port=3
  wires:
  x_ref/1 -> Sum/1
  x_vec/1 -> Sum/2
  Sum/1 -> Rate Transition/1
  Explicit_Robust_MPC_X/1 -> Bus Creator3/1, ReEnforceSaturation/1(u_ctrl)  "u_ctrl_x"
  Sum1/1 -> Rate Transition1/1
  y_ref/1 -> Sum1/1
  y_vec/1 -> Sum1/2
  Sum2/1 -> Rate Transition2/1
  z_ref/1 -> Sum2/1
  z_vec/1 -> Sum2/2
  ReEnforceSaturation/1(u_ctrl_out) -> Gain1/1
  Constant/1 -> ReEnforceSaturation/2(U_bounds)
  Explicit_Robust_MPC_Y/1 -> Bus Creator3/2, ReEnforceSaturation1/1(u_ctrl)  "u_ctrl_y"
  Constant1/1 -> ReEnforceSaturation1/2(U_bounds)
  Constant2/1 -> ReEnforceSaturation2/2(U_bounds)
  Explicit_Robust_MPC_Z/1 -> Bus Creator3/3, ReEnforceSaturation2/1(u_ctrl)  "u_ctrl_z"
  ReEnforceSaturation1/1(u_ctrl_out) -> Gain3/1
  ReEnforceSaturation2/1(u_ctrl_out) -> Gain5/1
  Explicit_Robust_MPC_X/2 -> Bus Creator/1  "flag_oob_x"
  Explicit_Robust_MPC_X/3 -> Bus Creator/2  "flag_minreg_x"
  Explicit_Robust_MPC_Y/2 -> Bus Creator1/1  "flag_oob_y"
  Explicit_Robust_MPC_Y/3 -> Bus Creator1/2  "flag_minreg_y"
  Explicit_Robust_MPC_Z/2 -> Bus Creator2/1  "flag_oob_z"
  Explicit_Robust_MPC_Z/3 -> Bus Creator2/2  "flag_minreg_z"
  Bus Creator3/1 -> Scope/1
  Bus Creator/1 -> Scope1/1
  Bus Creator1/1 -> Scope2/1
  Bus Creator2/1 -> Scope3/1
  Gain/1 -> Explicit_Robust_MPC_X/1
  Gain1/1 -> Rate Transition3/1
  Gain2/1 -> Explicit_Robust_MPC_Y/1
  Gain3/1 -> Rate Transition4/1
  Gain4/1 -> Explicit_Robust_MPC_Z/1
  Gain5/1 -> Rate Transition5/1
  Rate Transition/1 -> Gain/1
  Rate Transition1/1 -> Gain2/1
  Rate Transition2/1 -> Gain4/1
  Rate Transition4/1 -> u_ctrl_y/1
  Rate Transition3/1 -> u_ctrl_x/1
  Rate Transition5/1 -> Scope4/1, u_ctrl_z/1

== matlab function Rotate1/MATLAB Function1 ==
  data: u_ctrl_x input double; u_ctrl_y input double; u_ctrl_z input double; PolyRL_U2R parameter double; PolyT_U2R parameter double; TTR_mdl_Properties_arr parameter double; CA_M_X output double; CA_S_X output double; phi_ref output double; Ts_slow parameter double
function [CA_M_X,CA_S_X,phi_ref]  = Translation(u_ctrl_x,u_ctrl_y,u_ctrl_z, PolyRL_U2R,PolyT_U2R, TTR_mdl_Properties_arr , Ts_slow)
%#codegen

% TTR Properties
m_B    = TTR_mdl_Properties_arr(1);
g      = TTR_mdl_Properties_arr(2);
Ixx    = TTR_mdl_Properties_arr(3);
Iyy    = TTR_mdl_Properties_arr(4);
Izz    = TTR_mdl_Properties_arr(5);
Ixy    = TTR_mdl_Properties_arr(6);
Ixz    = TTR_mdl_Properties_arr(7);
Iyz    = TTR_mdl_Properties_arr(8);
d_RL_x = TTR_mdl_Properties_arr(9);
d_T_x  = TTR_mdl_Properties_arr(10);
d_RL_y = TTR_mdl_Properties_arr(11);
d_T_y  = TTR_mdl_Properties_arr(12);
d_RL_z = TTR_mdl_Properties_arr(13);
d_T_z  = TTR_mdl_Properties_arr(14);
h_RL   = TTR_mdl_Properties_arr(15);
h_T    = TTR_mdl_Properties_arr(16);
rho     = TTR_mdl_Properties_arr(17);
w_chord = TTR_mdl_Properties_arr(18);
w_span  = TTR_mdl_Properties_arr(19);
w_ac_x  = TTR_mdl_Properties_arr(20);
w_ac_y  = TTR_mdl_Properties_arr(21);


ca_m_right = PolyRL_U2R(1)*(u_ctrl_z/(2*(1+(d_RL_x/d_T_x)))); 
ca_m_left =  PolyRL_U2R(1)*(u_ctrl_z/(2*(1+(d_RL_x/d_T_x))));
ca_m_tail =  PolyT_U2R(1)*(u_ctrl_z*(1-1/(1+(d_RL_x/d_T_x))));

ca_s_right = u_ctrl_x;
ca_s_left = u_ctrl_x;
ca_s_tail = 0;

% Output
CA_M_X = [ca_m_right;ca_m_left;ca_m_tail];
CA_S_X = [ca_s_right;ca_s_left;ca_s_tail];
phi_ref = u_ctrl_y;

== matlab function MATLAB Function ==
  data: t input double; Theta input double; Theta_Dot input double; Theta_Die input double; CA_M_Theta output double; Theta_d input double; PolyRL_U2R parameter double; PolyT_U2R parameter double; CA_S_Theta output double; PolyGT_U2A parameter double; LQR_phi parameter double
function [CA_M_Theta,CA_S_Theta]  = Attitude(t, Theta,Theta_Dot,Theta_Die, Theta_d , PolyRL_U2R,PolyT_U2R,PolyGT_U2A , LQR_phi)
%#codegen

persistent t_km1;      if isempty(t_km1);      t_km1 = -0.02;      end;
persistent CA_M_Theta_km1; if isempty(CA_M_Theta_km1); CA_M_Theta_km1 = [0;0;0]; end;
persistent CA_S_Theta_km1; if isempty(CA_S_Theta_km1); CA_S_Theta_km1 = [0;0;0]; end;
persistent phi_err_int;  if isempty(phi_err_int);  phi_err_int = 0;  end;
persistent theta_err_int;  if isempty(theta_err_int);  theta_err_int = 0;  end;
persistent psi_err_int;  if isempty(psi_err_int);  psi_err_int = 0;  end;

Ts = 0.010;
if (t-t_km1 >= Ts)
    t_km1 = t;
    
% Gains
Ki_roll = 0;
Kp_roll_LU = [140 120 90];
Kd_roll = 17.5;
Kg_roll = 0.8;

Ki_pitch = 60;
Kp_pitch_LU = [190 170 140];
Kd_pitch = 22.5;
Kg_pitch = 1.25;

Ki_yaw = 60;
Kp_yaw = 300;
Kd_yaw = 150;
Kg_yaw = 0.0;

% Values
phi = Theta(1);
theta = Theta(2);
psi = Theta(3);
phi_dot = Theta_Dot(1);
theta_dot = Theta_Dot(2);
psi_dot = Theta_Dot(3);
phi_die = Theta_Die(1);
theta_die = Theta_Die(2);
psi_die = Theta_Die(3);

phi_d = Theta_d(1);
theta_d = Theta_d(2);
psi_d = Theta_d(3);


% Errors
phi_err = phi_d - phi;
phi_dot_err = 0 - phi_dot;
phi_die_err = 0 - phi_die;
theta_err = theta_d - theta;
theta_dot_err = 0 - theta_dot;
theta_die_err = 0 - theta_die;
psi_err = psi_d - psi;
psi_dot_err = 0 - psi_dot;
psi_die_err = 0 - psi_die;


% Ad-HOC
    Int_Leakage_Theta = 3.0;
    integrator_switch = 1;
    Yaw_Error_constraint = (pi/180)*( 20 );
    
    
% StateError Saturators
if ( psi_err < -Yaw_Error_constraint )
   psi_err = -Yaw_Error_constraint;
elseif ( psi_err > Yaw_Error_constraint )
   psi_err = Yaw_Error_constraint;
end


% StateError Integrators
    Phi_Error_Int_constraint = 1*(pi/180);   %[rad]
    Theta_Error_Int_constraint = 1*(pi/180);   %[rad]
    Psi_Error_Int_constraint = 1*(pi/180);   %[rad]
    Phi_Integrator_constraint = 10*(pi/180) * 3;  %[rad]*[s]
    Theta_Integrator_constraint = 10*(pi/180) * 3;  %[rad]*[s]
    Psi_Integrator_constraint = 10*(pi/180) * 3;  %[rad]*[s]
    a = (Ts/(Ts+2*Int_Leakage_Theta));

if integrator_switch == 0
    phi_err_int = 0;
    theta_err_int = 0;
    psi_err_int = 0;
else
if ( phi_err < -Phi_Error_Int_constraint )
  phi_err_intcnstr = -Phi_Error_Int_constraint;
elseif ( phi_err > Phi_Error_Int_constraint )
  phi_err_intcnstr = Phi_Error_Int_constraint;
else
  phi_err_intcnstr = phi_err;
end
if ( theta_err < -Theta_Error_Int_constraint )
  theta_err_intcnstr = -Theta_Error_Int_constraint;
elseif ( theta_err > Theta_Error_Int_constraint )
  theta_err_intcnstr = Theta_Error_Int_constraint;
else
  theta_err_intcnstr = theta_err;
end
if ( psi_err < -Psi_Error_Int_constraint )
  psi_err_intcnstr = -Psi_Error_Int_constraint;
elseif ( psi_err > Psi_Error_Int_constraint )
  psi_err_intcnstr = Psi_Error_Int_constraint;
else
  psi_err_intcnstr = psi_err;
end

if abs(phi_err_int) <= Phi_Integrator_constraint
    %phi_err_int = (1-a)*phi_err_int + phi_err*Ts;
    if (phi_d>phi  &&  phi_dot<=0*(pi/180))  ||  (phi_d<phi  &&  phi_dot>=-0*(pi/180))
        phi_err_int = phi_err_int + phi_err_intcnstr*Ts;
    end
    %phi_err_int = (1-a)*phi_err_int + a*(0);
elseif phi_err_int > Phi_Integrator_constraint  % !!! NOT >= , else the integrated value gets stuck w/o LP leakage
    phi_err_int = Phi_Integrator_constraint;
elseif phi_err_int < -Phi_Integrator_constraint  % !!! NOT <= , else the integrated value gets stuck w/o LP leakage
    phi_err_int = -Phi_Integrator_constraint;
end
if abs(theta_err_int) <= Theta_Integrator_constraint
    %theta_err_int = (1-a)*theta_err_int + theta_err*Ts;
    if (theta_d>theta  &&  theta_dot<=0*(pi/180))  ||  (theta_d<theta  &&  theta_dot>=-0*(pi/180))
        theta_err_int = theta_err_int + theta_err_intcnstr*Ts;
    end
    %theta_err_int = (1-a)*theta_err_int + a*(0);
elseif theta_err_int > Theta_Integrator_constraint  % !!! NOT >= , else the integrated value gets stuck w/o LP leakage
    theta_err_int = Theta_Integrator_constraint;
elseif theta_err_int < -Theta_Integrator_constraint  % !!! NOT <= , else the integrated value gets stuck w/o LP leakage
    theta_err_int = -Theta_Integrator_constraint;
end  
if abs(psi_err_int) <= Psi_Integrator_constraint
    %psi_err_int = (1-a)*psi_err_int + psi_err*Ts;
    if (psi_d>psi  &&  psi_dot<=0*(pi/180))  ||  (psi_d<psi  &&  psi_dot>=-0*(pi/180))
        psi_err_int = psi_err_int + psi_err_intcnstr*Ts;
    end
    %psi_err_int = (1-a)*psi_err_int + a*(0);
elseif psi_err_int > Psi_Integrator_constraint  % !!! NOT >= , else the integrated value gets stuck w/o LP leakage
    psi_err_int = Psi_Integrator_constraint;
elseif psi_err_int < -Psi_Integrator_constraint  % !!! NOT <= , else the integrated value gets stuck w/o LP leakage
    psi_err_int = -Psi_Integrator_constraint;
end
end


% Control
LUx = (pi/180)*([0 5 10]);  %[rad]
Kp_roll = interp1(LUx,Kp_roll_LU, abs(phi_err) ,'linear',Kp_roll_LU(length(Kp_roll_LU)));
if Kp_roll < 0;  Kp_roll = 0;  end;
Kp_pitch = interp1(LUx,Kp_pitch_LU, abs(theta_err) ,'linear',Kp_pitch_LU(length(Kp_pitch_LU)));
if Kp_pitch < 0;  Kp_pitch = 0;  end;


roll_control = Ki_roll*phi_err_int + Kp_roll*phi_err + Kd_roll*phi_dot_err + Kg_roll*phi_die_err;  %[us]
pitch_control = Ki_pitch*theta_err_int + Kp_pitch*theta_err + Kd_pitch*theta_dot_err + Kg_pitch*theta_die_err;  %[us]
yaw_control = Ki_yaw*psi_err_int + Kp_yaw*psi_err + Kd_yaw*psi_dot_err + Kg_yaw*psi_die_err;

PHI_ctrl = [phi_err_int; phi_err; phi_dot_err; phi_die_err; 0];
roll_control = [Ki_roll LQR_phi] * PHI_ctrl;  %[us]


ca_m_right = PolyRL_U2R(1)*(-roll_control + pitch_control); 
ca_m_left =  PolyRL_U2R(1)*(roll_control + pitch_control);
ca_m_tail =  PolyT_U2R(1)*(-pitch_control);

ca_s_right = 0;
ca_s_left = 0;
ca_s_tail = PolyGT_U2A(1)*(-yaw_control);

% Output
CA_M_Theta = [ca_m_right;ca_m_left;ca_m_tail];
CA_S_Theta = [ca_s_right;ca_s_left;ca_s_tail];

CA_M_Theta_km1 = CA_M_Theta;
CA_S_Theta_km1 = CA_S_Theta;

else
  CA_M_Theta = CA_M_Theta_km1;
  CA_S_Theta = CA_S_Theta_km1;
end;

== matlab function MATLAB Function2 ==
  data: y output double; t input double; u input double
function y  = slew(t,u)
%#codegen

persistent t_km1; if isempty(t_km1); t_km1 = -0.02;  end;
persistent y_km1; if isempty(y_km1); y_km1 = u;  end;

Ts = 0.01;
if (t-t_km1 >= Ts)
    t_km1 = t;

slewrate = (5*(pi/180))*Ts;

y = u;
if u - y_km1 > slewrate
    y = y_km1 + slewrate;
elseif u - y_km1 < -slewrate
    y = y_km1 - slewrate;
end

y_km1 = y;

else
    
y = y_km1;

end

== matlab function Rotate1/TTR_RobustMPC/ReEnforceSaturation ==
  data: u_ctrl input double; u_ctrl_out output double; U_bounds input double
function u_ctrl_out = ReEnforceSaturations(u_ctrl,U_bounds)
%#codegen

%   this block enforces again the control action saturations. It is not
%   needed and it has been verified that it is not needed. But... you never
%   know. It is always relaxing to be sure that the saturators are enforced
%   whatsoever

u_ctrl_out = u_ctrl;

if length(u_ctrl) ~= (length(U_bounds)/2)
    % that can't be valid! 
    u_ctrl_out = 0; % do something meaningfull hoping that we will save the system...
    flag_inconsistency = 1; % inform the user...
else
    % ok all fine...
    for i = 1:length(u_ctrl)
        u_ctrl_out(i) = max(u_ctrl(i),U_bounds(2*(i-1)+1));
        u_ctrl_out(i) = min(u_ctrl(i),U_bounds(2*(i-1)+2));
    end
end

end

== matlab function Rotate1/TTR_RobustMPC/ReEnforceSaturation1 ==
  data: u_ctrl input double; u_ctrl_out output double; U_bounds input double
function u_ctrl_out = ReEnforceSaturations(u_ctrl,U_bounds)
%#codegen

%   this block enforces again the control action saturations. It is not
%   needed and it has been verified that it is not needed. But... you never
%   know. It is always relaxing to be sure that the saturators are enforced
%   whatsoever

u_ctrl_out = u_ctrl;

if length(u_ctrl) ~= (length(U_bounds)/2)
    % that can't be valid! 
    u_ctrl_out = 0; % do something meaningfull hoping that we will save the system...
    flag_inconsistency = 1; % inform the user...
else
    % ok all fine...
    for i = 1:length(u_ctrl)
        u_ctrl_out(i) = max(u_ctrl(i),U_bounds(2*(i-1)+1));
        u_ctrl_out(i) = min(u_ctrl(i),U_bounds(2*(i-1)+2));
    end
end

end

== matlab function Rotate1/TTR_RobustMPC/ReEnforceSaturation2 ==
  data: u_ctrl input double; u_ctrl_out output double; U_bounds input double
function u_ctrl_out = ReEnforceSaturations(u_ctrl,U_bounds)
%#codegen

%   this block enforces again the control action saturations. It is not
%   needed and it has been verified that it is not needed. But... you never
%   know. It is always relaxing to be sure that the saturators are enforced
%   whatsoever

u_ctrl_out = u_ctrl;

if length(u_ctrl) ~= (length(U_bounds)/2)
    % that can't be valid! 
    u_ctrl_out = 0; % do something meaningfull hoping that we will save the system...
    flag_inconsistency = 1; % inform the user...
else
    % ok all fine...
    for i = 1:length(u_ctrl)
        u_ctrl_out(i) = max(u_ctrl(i),U_bounds(2*(i-1)+1));
        u_ctrl_out(i) = min(u_ctrl(i),U_bounds(2*(i-1)+2));
    end
end

end

== matlab function Rotate/rotate_IMU_2_LTP ==
  data: phi_dot output double; theta_dot output double; psi_dot output double; x_dot output double; Theta_in input double; y_dot output double; z_dot output double; phi_die output double; theta_die output double; psi_die output double; x_die output double; y_die output double; z_die output double; X_in input double; Omega_in input double; U_in input double; Omega_Dot_in input double; U_Dot_in input double
function [phi_dot,theta_dot,psi_dot,x_dot,y_dot,z_dot,phi_die,theta_die,psi_die,x_die,y_die,z_die] = rotate_IMU_2_LTP(Theta_in,X_in,Omega_in,U_in,Omega_Dot_in,U_Dot_in)
%#codegen


% Theta is already in LTP coordinate frame
Theta = Theta_in;  %phi,theta,psi

% Rotate U to LTP
X_Dot = Rotate_IMUframe_2_Frame(U_in,Theta(1),Theta(2),0);  %FORCE yaw rotation to 0

% Rotate U_Dot to LTP
X_Die = Rotate_IMUframe_2_Frame(U_Dot_in,Theta(1),Theta(2),0);  %FORCE yaw rotation to 0

% Rotate Omega to LTP
Theta_Dot = Rotate_IMUrates_2_Frame(Omega_in,Theta(1),Theta(2));

% Rotate Omega_Dot to LTP
Theta_Die = Rotate_IMUrates_2_Frame(Omega_Dot_in,Theta(1),Theta(2));


phi_dot = Theta_Dot(1);
theta_dot = Theta_Dot(2);
psi_dot = Theta_Dot(3);
x_dot = X_Dot(1);
y_dot = X_Dot(2);
z_dot = X_Dot(3);
phi_die = Theta_Die(1);
theta_die = Theta_Die(2);
psi_die = Theta_Die(3);
x_die = X_Die(1);
y_die = X_Die(2);
z_die = X_Die(3);
